simulink model "statechart"  (R2024b)
settings: Solver=FixedStepDiscrete  StartTime=0.0  StopTime=60  FixedStep=1  RelTol=1e-3
libraries: simulink x2, SignalEditorBlockLib x1
settings Model: PacingRate=9  Creator=adetunji  LastModifiedBy=adetunji
settings ConfigComp: CovEnable=on  RecordCoverage=on  CovModelRefEnable=on

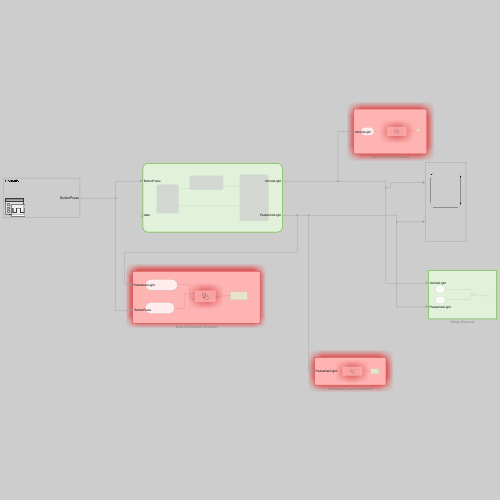
[thumbnail: Simulink's stored preview of the top-level diagram]
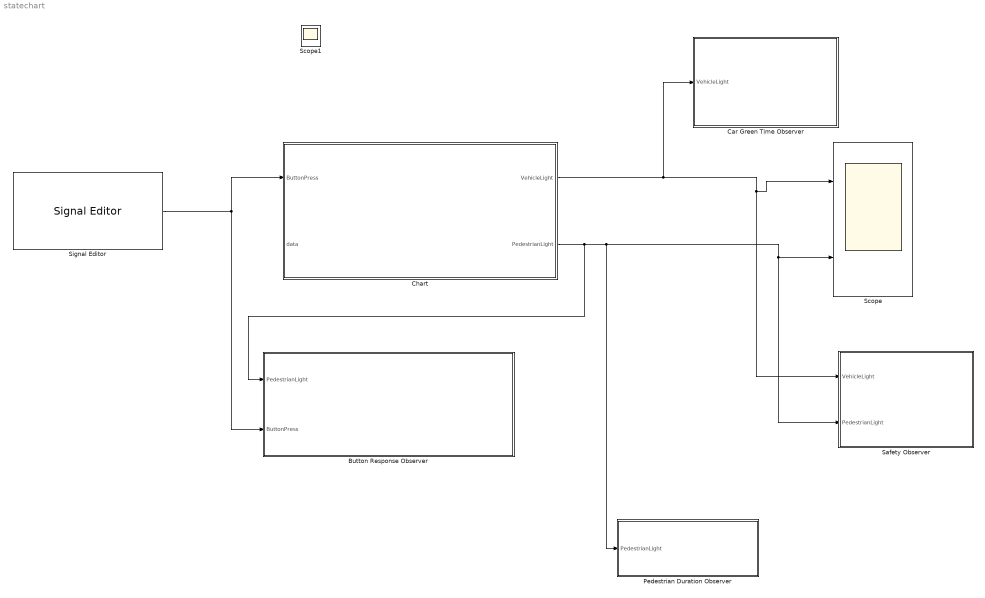
== system statechart ==
  Button Response Observer : Subsystem
  Car Green Time Observer : Subsystem
  Chart : Stateflow chart  TreatAsAtomicUnit=on
  Pedestrian Duration Observer : Subsystem
  Safety Observer : Subsystem
  Scope : Scope  NumInputPorts=2
  Signal Editor : SignalEditorBlockLib/Signal Editor  FileName=ButtonPress.mat  ActiveScenario=Scenario  ActiveSignal=ButtonPress  IsBus=off  OutputBusObjectStr=Bus: BusObject  SampleTime=0  Interpolate=off  ZeroCross=off  OutputAfterFinalValue=Setting to zero  Unit=inherit  PreserveSignalName=on  ApplySigPropsToAllScenarios=on  ApplySigPropsToAllSignals=off
  Scope1 : Scope
  wires:
  Chart/1(VehicleLight) -> Car Green Time Observer/1(VehicleLight), Safety Observer/1(VehicleLight), Scope/1
  Signal Editor/1 -> Button Response Observer/2(" ButtonPress"), Chart/1(ButtonPress)
  Chart/2(PedestrianLight) -> Button Response Observer/1(PedestrianLight), Pedestrian Duration Observer/1(PedestrianLight), Safety Observer/2(PedestrianLight), Scope/2

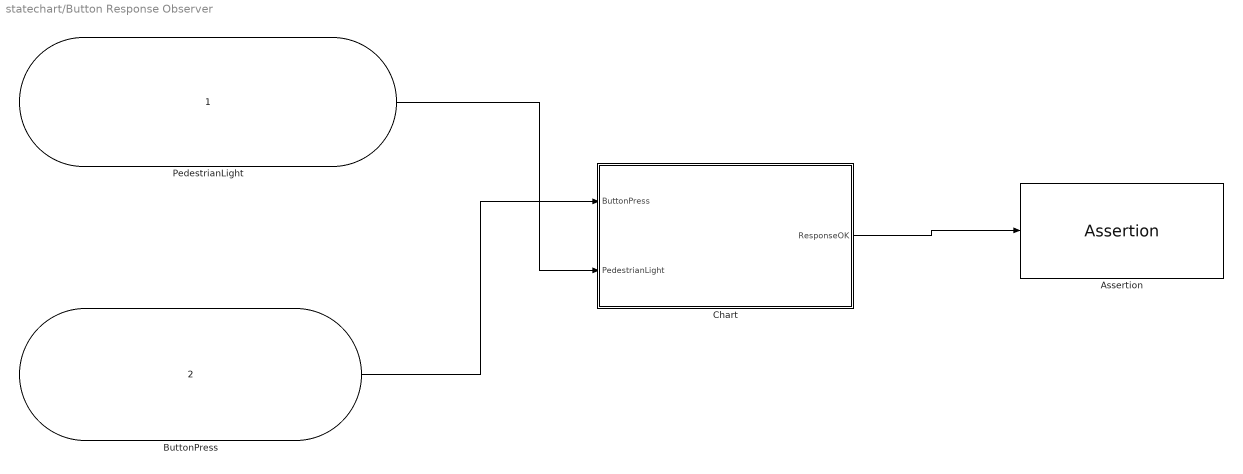
== system statechart/Button Response Observer ==
  PedestrianLight : Inport
  " ButtonPress" : Inport  Port=2
  Assertion : Assertion
  Chart : Stateflow chart  TreatAsAtomicUnit=on
  wires:
  " ButtonPress"/1 -> Chart/1(ButtonPress)
  PedestrianLight/1 -> Chart/2(PedestrianLight)
  Chart/1(ResponseOK) -> Assertion/1

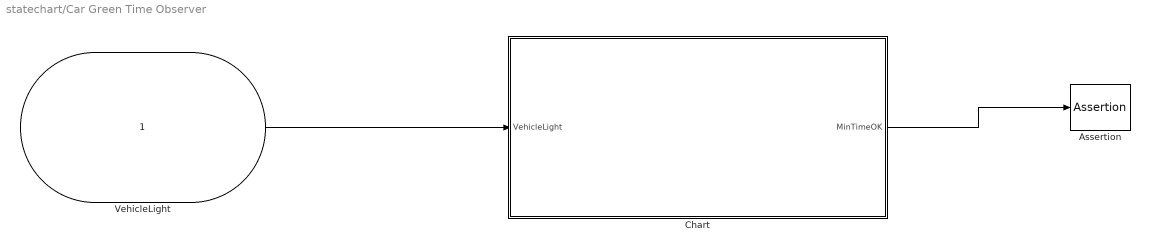
== system statechart/Car Green Time Observer ==
  VehicleLight : Inport
  Assertion : Assertion
  Chart : Stateflow chart  TreatAsAtomicUnit=on
  wires:
  VehicleLight/1 -> Chart/1(VehicleLight)
  Chart/1(MinTimeOK) -> Assertion/1

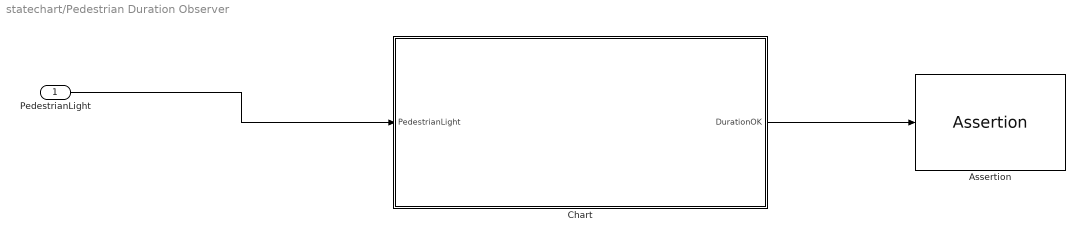
== system statechart/Pedestrian Duration Observer ==
  PedestrianLight : Inport
  Assertion : Assertion
  Chart : Stateflow chart  TreatAsAtomicUnit=on
  wires:
  Chart/1(DurationOK) -> Assertion/1
  PedestrianLight/1 -> Chart/1(PedestrianLight)

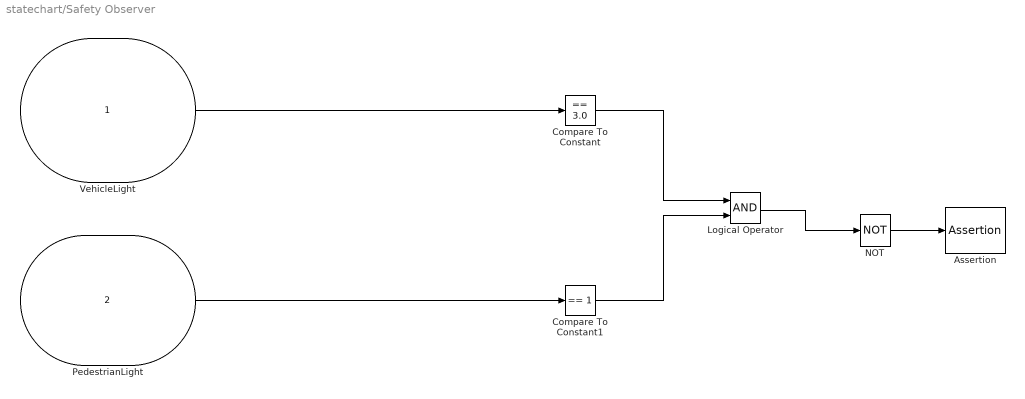
== system statechart/Safety Observer ==
  VehicleLight : Inport
  PedestrianLight : Inport  Port=2
  Assertion : Assertion
  Compare To Constant : simulink/Logic and Bit Operations/Compare To Constant  relop===  const=3.0  OutDataTypeStr=boolean
  Compare To Constant1 : simulink/Logic and Bit Operations/Compare To Constant  relop===  const=1  OutDataTypeStr=boolean
  Logical Operator : Logic  AllPortsSameDT=off  OutDataTypeStr=boolean
  NOT : Logic  Operator=NOT  IconShape=distinctive  AllPortsSameDT=off  OutDataTypeStr=boolean
  wires:
  VehicleLight/1 -> Compare To Constant/1
  PedestrianLight/1 -> Compare To Constant1/1
  Compare To Constant/1 -> Logical Operator/1
  Compare To Constant1/1 -> Logical Operator/2
  Logical Operator/1 -> NOT/1
  NOT/1 -> Assertion/1

== stateflow chart statechart/Car Green Time Observer/Chart ==
  state NotGreen
    entry: MinTimeOK = 1;
  state GreenTiming
    entry: MinTimeOK = 1;
  (default) -> NotGreen
  NotGreen -> GreenTiming : [VehicleLight == 3]
  GreenTiming -> NotGreen [order 1] : [VehicleLight ~= 3 && after(10,sec)]
  GreenTiming -> NotGreen [order 2] : [VehicleLight ~= 3 && ~after(10,sec)] /{ MinTimeOK = 0;}
  data: VehicleLight input size=1; MinTimeOK output size=1 =1

== stateflow chart statechart/Button Response Observer/Chart ==
  state Idle
    entry: ResponseOK = 1;
  state WaitingForGreen
    entry: ResponseOK = 1;
  state CheckTiming
    entry: ResponseOK = 1;
    during: if PedestrianLight == 1; ResponseOK = 1; else; ResponseOK = 0; end
  (default) -> Idle
  Idle -> WaitingForGreen : [ButtonPress == 1]
  WaitingForGreen -> CheckTiming [order 1] : after(18,sec)
  WaitingForGreen -> Idle [order 2] : [PedestrianLight == 1]
  CheckTiming -> Idle : [PedestrianLight == 1 || after(1,sec)]
  data: ButtonPress input size=1; PedestrianLight input size=1; ResponseOK output size=1 =1

== stateflow chart statechart/Chart ==
  state Crossing
    entry: VehicleLight = 1; PedestrianLight = 1;
  state Amber
    entry: VehicleLight = 2; PedestrianLight = 0;
  state Idle
    entry: VehicleLight = 3; PedestrianLight = 0;
  (default) -> Idle
  Amber -> Crossing : after(3,sec)
  Idle -> Amber : [ButtonPress == 1]
  Crossing -> Idle : after(15,sec)
  data: ButtonPress input size=1; VehicleLight output size=1; PedestrianLight output size=1; data input

== stateflow chart statechart/Pedestrian Duration Observer/Chart ==
  state NotGreen
    entry: DurationOK = 1;
  state TimingGreen
    entry: DurationOK = 1;
  (default) -> NotGreen
  NotGreen -> TimingGreen : [PedestrianLight == 1]
  TimingGreen -> NotGreen [order 2] : [PedestrianLight == 0 && after(15,sec)]
  TimingGreen -> NotGreen [order 1] : [PedestrianLight == 0 && ~after(15,sec)] /{ DurationOK = 0;}
  data: PedestrianLight input size=1; DurationOK output size=1 =1
